simulink model "Component"  (R2024a)
settings: Solver=VariableStepAuto  StartTime=0.0  StopTime=10.0  RelTol=1e-3
undefined symbols (not defined in the file or in its folder): canChannel
libraries: canmsglib x3, canlib x2
settings Model: DataDictionary=BMS_System_dict1.sldd  Creator=hirah  LastModifiedBy=hirah

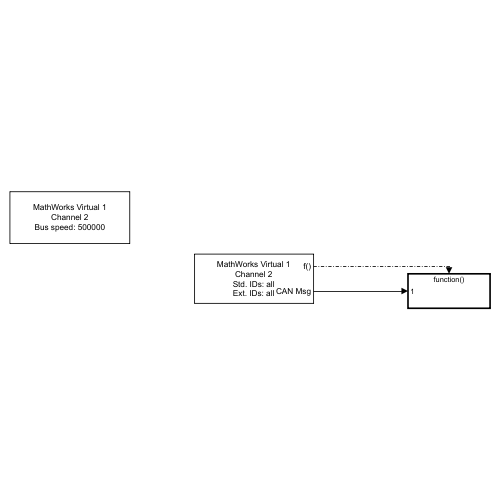
[thumbnail: Simulink's stored preview of the top-level diagram]
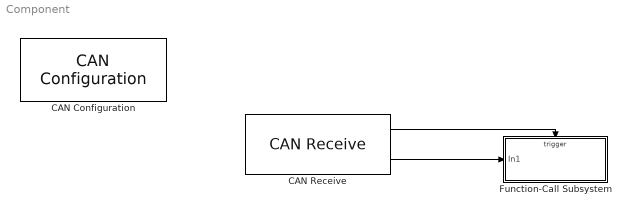
== system Component ==
  CAN Configuration : canlib/CAN Configuration  BlockHandle=585.0005  Device=MathWorks Virtual 1 (Channel 2)  DeviceMenu=MathWorks Virtual 1 (Channel 2)  ObjConstructor=canChannel('MathWorks', 'Virtual 1', 2)  BusSpeed=500000  EnableBitParameters=off  AckMode=Normal
  CAN Receive : canlib/CAN Receive  BlockHandle=586.0002  Device=MathWorks Virtual 1 (Channel 2)  DeviceMenu=MathWorks Virtual 1 (Channel 2)  ObjConstructor=canChannel('MathWorks', 'Virtual 1', 2)  EnableStandardIDsFilter=off  StdIDsCombo=Allow all  StandardIDs=261  EnableExtendedIDsFilter=off  ExtIDsCombo=Allow all  ExtendedIDs=0  SampleTime=0.01  MsgsPerTimestep=all  InternalFilterUpdateStatus=on  BusOutput=off
  Function-Call Subsystem : Subsystem  TreatAsAtomicUnit=on
  wires:
  CAN Receive/1 -> Function-Call Subsystem/Trigger
  CAN Receive/2 -> Function-Call Subsystem/1(In1)

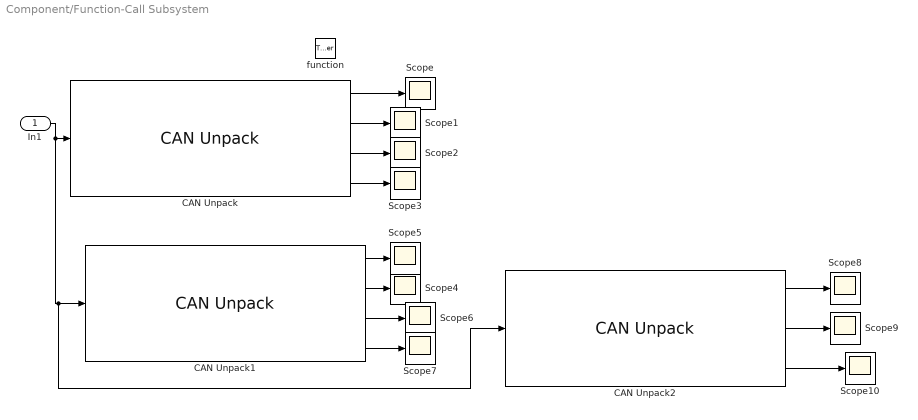
== system Component/Function-Call Subsystem ==
  In1 : Inport
  function : TriggerPort  TriggerType=function-call  VariantControl=(inherit)
  CAN Unpack : canmsglib/CAN Unpack  CANdbFile=C:\Users\hirah\Downloads\BMS_CAN_Database (5).dbc  MsgList=frmPackMeasurements  MsgName=frmPackMeasurements  MsgIDType=Standard (11-bit identifier)  MsgIdentifier=256  MsgLength=6  SignalInfo={ 'sigPackCurrent', '16', '16', 'LE', 'signed', 'Standard', '0', '0.1', '0', '-400', '400'; 'sigPackTempAvg', '32', '8', 'LE', 'unsigned', 'Standard', '0', '1', '-40', '-40', '150'; 'sigPackTempMax', '40', '8', 'LE', 'unsigned', 'Standard', '0', '1', '-40', '-40', '150'; 'sigPackVoltage', '0', '16', 'LE', 'unsigned', 'Standard', '0', '0.1', '0', '0', '1000' }  IDPort=off  TimestampPort=off  ErrorPort=off  RemotePort=off  LengthPort=off  StatusPort=off  ApplyMinMax=off
      settings: DataFormat=CANdb specified signals
  CAN Unpack1 : canmsglib/CAN Unpack  CANdbFile=C:\Users\hirah\Downloads\BMS_CAN_Database (5).dbc  MsgList=frmBMSStateEstimation  MsgName=frmBMSStateEstimation  MsgIDType=Standard (11-bit identifier)  MsgIdentifier=259  MsgLength=6  SignalInfo={ 'sigSOC', '0', '8', 'LE', 'unsigned', 'Standard', '0', '1', '0', '0', '100'; 'sigSOH', '8', '8', 'LE', 'unsigned', 'Standard', '0', '1', '0', '0', '100'; 'sigSOPCharge', '32', '16', 'LE', 'unsigned', 'Standard', '0', '1', '0', '0', '200'; 'sigSOPDischarge', '16', '16', 'LE', 'unsigned', 'Standard', '0', '1', '0', '0', '200' }  IDPort=off  TimestampPort=off  ErrorPort=off  RemotePort=off  LengthPort=off  StatusPort=off  ApplyMinMax=off
      settings: DataFormat=CANdb specified signals
  CAN Unpack2 : canmsglib/CAN Unpack  CANdbFile=C:\Users\hirah\Downloads\BMS_CAN_Database (5).dbc  MsgList=frmSensorHealth  MsgName=frmSensorHealth  MsgIDType=Standard (11-bit identifier)  MsgIdentifier=258  MsgLength=3  SignalInfo={ 'sigCurrentSensorsStatus', '8', '8', 'LE', 'unsigned', 'Standard', '0', '1', '0', '0', '3'; 'sigTempSensorsStatus', '16', '8', 'LE', 'unsigned', 'Standard', '0', '1', '0', '0', '3'; 'sigVoltageSensorsStatus', '0', '8', 'LE', 'unsigned', 'Standard', '0', '1', '0', '0', '3' }  IDPort=off  TimestampPort=off  ErrorPort=off  RemotePort=off  LengthPort=off  StatusPort=off  ApplyMinMax=off
      settings: DataFormat=CANdb specified signals
  Scope{,1..10} (11 alike) : Scope
  wires:
  In1/1 -> CAN Unpack2/1, CAN Unpack1/1, CAN Unpack/1
  CAN Unpack/1 -> Scope/1
  CAN Unpack/4 -> Scope3/1
  CAN Unpack/3 -> Scope2/1
  CAN Unpack/2 -> Scope1/1
  CAN Unpack1/2 -> Scope4/1
  CAN Unpack1/1 -> Scope5/1
  CAN Unpack1/3 -> Scope6/1
  CAN Unpack1/4 -> Scope7/1
  CAN Unpack2/1 -> Scope8/1
  CAN Unpack2/3 -> Scope10/1
  CAN Unpack2/2 -> Scope9/1
